simulink model "Final_V620140905h5b_fuben1"  (Simulink 7.9)
settings: Solver=FixedStepDiscrete  StartTime=0.0  StopTime=1  FixedStep=Auto  RelTol=1e-3
undefined symbols (not defined in the file or in its folder): Down, Up
libraries: tiiqmathlib x157, idelinklib_common x83, c2833xlib x37, simulink x12, c28xdmclib x12, c280xlib x7, simulink_extras x4, commutil2 x2, idelinklib_tgtpref x1, idelinklib_ticcs x1
(part 5 of 7)

== system Final_V620140905h5b_fuben1/Function-Call Subsystem1/RC filter2 ==
  x : Inport
  Constant2 : Constant  Value=a  OutDataTypeStr=fixdt(1,32,16)
  Constant3 : Constant  Value=1-a  OutDataTypeStr=fixdt(1,32,16)
  IQN x IQN : tiiqmathlib/IQN x IQN  multiplyOption=Multiply
  IQN x IQN1 : tiiqmathlib/IQN x IQN  multiplyOption=Multiply
  Sum2 : Sum
  Unit Delay2 : UnitDelay  SampleTime=-1
  y : Outport
  wires:
  x/1 -> IQN x IQN/1
  Constant2/1 -> IQN x IQN/2
  Constant3/1 -> IQN x IQN1/1
  IQN x IQN/1 -> Sum2/1
  IQN x IQN1/1 -> Sum2/2
  Sum2/1 -> y/1, Unit Delay2/1
  Unit Delay2/1 -> IQN x IQN1/2

== system Final_V620140905h5b_fuben1/Function-Call Subsystem1/RC filter3 ==
  x : Inport
  Constant2 : Constant  Value=a  OutDataTypeStr=Inherit: Inherit via back propagation
  Constant3 : Constant  Value=1-a  OutDataTypeStr=Inherit: Inherit via back propagation
  IQN x IQN : tiiqmathlib/IQN x IQN  multiplyOption=Multiply
  IQN x IQN1 : tiiqmathlib/IQN x IQN  multiplyOption=Multiply
  Sum2 : Sum
  Unit Delay2 : UnitDelay  SampleTime=-1
  y : Outport
  wires:
  Unit Delay2/1 -> IQN x IQN1/2
  Sum2/1 -> Unit Delay2/1, y/1
  IQN x IQN1/1 -> Sum2/2
  IQN x IQN/1 -> Sum2/1
  Constant3/1 -> IQN x IQN1/1
  Constant2/1 -> IQN x IQN/2
  x/1 -> IQN x IQN/1

== system Final_V620140905h5b_fuben1/Function-Call Subsystem1/RC filter4 ==
  x : Inport
  Constant2 : Constant  Value=a  OutDataTypeStr=Inherit: Inherit via back propagation
  Constant3 : Constant  Value=1-a  OutDataTypeStr=Inherit: Inherit via back propagation
  IQN x IQN : tiiqmathlib/IQN x IQN  multiplyOption=Multiply
  IQN x IQN1 : tiiqmathlib/IQN x IQN  multiplyOption=Multiply
  Sum2 : Sum
  Unit Delay2 : UnitDelay  SampleTime=-1
  y : Outport
  wires:
  x/1 -> IQN x IQN/1
  Constant2/1 -> IQN x IQN/2
  Constant3/1 -> IQN x IQN1/1
  IQN x IQN/1 -> Sum2/1
  IQN x IQN1/1 -> Sum2/2
  Sum2/1 -> y/1, Unit Delay2/1
  Unit Delay2/1 -> IQN x IQN1/2

== system Final_V620140905h5b_fuben1/Function-Call Subsystem1/RC filter9 ==
  x : Inport
  Constant2 : Constant  Value=a  OutDataTypeStr=fixdt(1,32,16)
  Constant3 : Constant  Value=1-a  OutDataTypeStr=fixdt(1,32,16)
  IQN x IQN : tiiqmathlib/IQN x IQN  multiplyOption=Multiply
  IQN x IQN1 : tiiqmathlib/IQN x IQN  multiplyOption=Multiply
  Sum2 : Sum
  Unit Delay2 : UnitDelay  SampleTime=-1
  y : Outport
  wires:
  Unit Delay2/1 -> IQN x IQN1/2
  Sum2/1 -> Unit Delay2/1, y/1
  IQN x IQN1/1 -> Sum2/2
  IQN x IQN/1 -> Sum2/1
  Constant3/1 -> IQN x IQN1/1
  Constant2/1 -> IQN x IQN/2
  x/1 -> IQN x IQN/1

== system Final_V620140905h5b_fuben1/Function-Call Subsystem1/Soft-start1 ==
  Reset : Inport
  Constant29 : Constant  Value=a  OutDataTypeStr=fixdt(1,32,16)
  Integration 0 to maximal1 : Subsystem
  Vref : Outport
  wires:
  Reset/1 -> Integration 0 to maximal1/2(Reset)
  Integration 0 to maximal1/1(y) -> Vref/1
  Constant29/1 -> Integration 0 to maximal1/1(x)

== system Final_V620140905h5b_fuben1/Function-Call Subsystem1/Soft-start2 ==
  Reset : Inport
  Constant29 : Constant  Value=a  OutDataTypeStr=fixdt(1,32,16)
  Integration 0 to maximal1 : Subsystem
  Vref : Outport
  wires:
  Constant29/1 -> Integration 0 to maximal1/1(x)
  Integration 0 to maximal1/1(y) -> Vref/1
  Reset/1 -> Integration 0 to maximal1/2(Reset)

== system Final_V620140905h5b_fuben1/Function-Call Subsystem1/Soft-start4 ==
  Reset : Inport
  T : Inport  Port=2
  Constant9 : Constant  Value=0.01  OutDataTypeStr=fixdt(1,32,16)
  IQN / IQN : tiiqmathlib/IQN // IQN
  Integration 0 to maximal1 : Subsystem
  Vref : Outport
  wires:
  Reset/1 -> Integration 0 to maximal1/2(Reset)
  Integration 0 to maximal1/1(y) -> Vref/1
  Constant9/1 -> IQN / IQN/1
  IQN / IQN/1 -> Integration 0 to maximal1/1(x)
  T/1 -> IQN / IQN/2

== system Final_V620140905h5b_fuben1/Function-Call Subsystem1/Soft-start5 ==
  Reset : Inport
  Constant29 : Constant  Value=a  OutDataTypeStr=fixdt(1,32,16)
  Integration 0 to maximal1 : Subsystem
  Vref : Outport
  wires:
  Reset/1 -> Integration 0 to maximal1/2(Reset)
  Integration 0 to maximal1/1(y) -> Vref/1
  Constant29/1 -> Integration 0 to maximal1/1(x)

== system Final_V620140905h5b_fuben1/Function-Call Subsystem1/Soft-start6 ==
  Reset : Inport
  Constant29 : Constant  Value=a  OutDataTypeStr=fixdt(1,32,16)
  Integration 0 to maximal1 : Subsystem
  Vref : Outport
  wires:
  Reset/1 -> Integration 0 to maximal1/2(Reset)
  Integration 0 to maximal1/1(y) -> Vref/1
  Constant29/1 -> Integration 0 to maximal1/1(x)

== system Final_V620140905h5b_fuben1/Function-Call Subsystem1/Soft_turn_off ==
  In : Inport
  Enable : Inport  Port=2
  Constant5 : Constant  Value=0.5  OutDataTypeStr=fixdt(1,32,16)
  Saturation1 : Saturate  UpperLimit=1000  LowerLimit=0  LinearizeAsGain=off  ZeroCross=off  OutDataTypeStr=fixdt(1,32,16)
  Sum1 : Sum  Inputs=+-
  Switch4 : Switch  Criteria=u2 > Threshold  SaturateOnIntegerOverflow=on  InputSameDT=on
  Switch5 : Switch  Criteria=u2 > Threshold  SaturateOnIntegerOverflow=on  InputSameDT=on
  Unit Delay2 : UnitDelay  SampleTime=-1
  Ref : Outport
  wires:
  In/1 -> Switch5/1, Switch4/1
  Switch4/1 -> Ref/1
  Constant5/1 -> Sum1/2
  Unit Delay2/1 -> Sum1/1
  Sum1/1 -> Switch5/3
  Switch5/1 -> Saturation1/1
  Enable/1 -> Switch5/2, Switch4/2
  Saturation1/1 -> Switch4/3, Unit Delay2/1

== system Final_V620140905h5b_fuben1/Function-Call Subsystem1/Soft_turn_on ==
  Enable : Inport
  Vdc : Inport  Port=2
  Compare To Constant2 : simulink/Logic and Bit Operations/Compare To Constant  relop=>  const=165*0.97/1.732  OutDataTypeStr=boolean
  Logical Operator5 : Logic  AllPortsSameDT=off  OutDataTypeStr=boolean
  Relay1 : Relay  OnSwitchValue=680  OffSwitchValue=650  OutDataTypeStr=Inherit: Inherit via back propagation
  Sum16 : Sum
  Voltage soft start (from 0 to 1 within 10s)1 : Subsystem  mask{a=10, b=401/1.732, c=0}
      mask prompts: a "soft time"; b "max limit"; c "min limit"
  Voltage soft start (from 0 to 120 within 5s) : Subsystem  mask{a=10, b=165/1.732, c=0}
      mask prompts: a "soft time"; b "max limit"; c "min limit"
  Out : Outport
  wires:
  Voltage soft start (from 0 to 120 within 5s)/1(k) -> Sum16/1, Compare To Constant2/1
  Enable/1 -> Voltage soft start (from 0 to 120 within 5s)/1(Reset)
  Sum16/1 -> Out/1
  Vdc/1 -> Relay1/1
  Compare To Constant2/1 -> Logical Operator5/1
  Voltage soft start (from 0 to 1 within 10s)1/1(k) -> Sum16/2
  Logical Operator5/1 -> Voltage soft start (from 0 to 1 within 10s)1/1(Reset)
  Relay1/1 -> Logical Operator5/2

== system Final_V620140905h5b_fuben1/Function-Call Subsystem1/Subsystem ==
  Trig : Inport
  x : Inport  Port=2
  Constant11 : Constant  Value=30  OutDataTypeStr=fixdt(1,32,16)
  Constant7 : Constant  Value=50  OutDataTypeStr=fixdt(1,32,16)
  Relational Operator1 : RelationalOperator
  Relational Operator2 : RelationalOperator  Operator=<=
  Saturation2 : Saturate  UpperLimit=500  LowerLimit=-500  LinearizeAsGain=off  ZeroCross=off  OutDataTypeStr=fixdt(1,32,16)
  Triggered Subsystem1 : Subsystem  TreatAsAtomicUnit=on
  sample per n times : Subsystem  mask{n=200*10}
      mask prompts: n "Counter time n"
  On/off : Outport
  sum : Outport  Port=2
  wires:
  Constant11/1 -> Relational Operator1/1
  sample per n times/1(sum) -> Saturation2/1
  Triggered Subsystem1/1(Count1) -> Relational Operator2/2
  Constant7/1 -> Relational Operator2/1
  Relational Operator1/1 -> Triggered Subsystem1/1(Reset1)
  Trig/1 -> Triggered Subsystem1/Trigger
  Relational Operator2/1 -> On/off/1
  x/1 -> sample per n times/1(x)
  Saturation2/1 -> Relational Operator1/2, sum/1

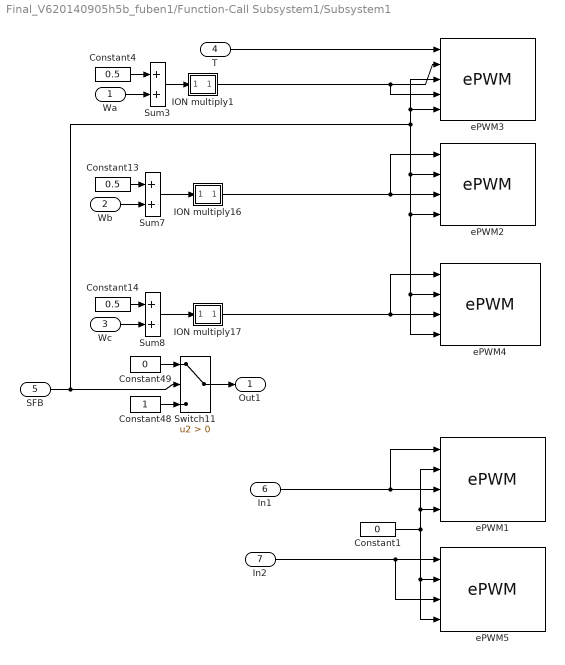
== system Final_V620140905h5b_fuben1/Function-Call Subsystem1/Subsystem1 ==
  Wa : Inport
  Wb : Inport  Port=2
  Wc : Inport  Port=3
  T : Inport  Port=4
  SFB : Inport  Port=5
  In1 : Inport  Port=6
  In2 : Inport  Port=7
  Constant1 : Constant  Value=0  OutDataTypeStr=fixdt(1,32,16)
  Constant13 : Constant  Value=0.5  OutDataTypeStr=fixdt(1,32,16)
  Constant14 : Constant  Value=0.5  OutDataTypeStr=fixdt(1,32,16)
  Constant4 : Constant  Value=0.5  OutDataTypeStr=fixdt(1,32,16)
  Constant48 : Constant  OutDataTypeStr=int16
  Constant49 : Constant  Value=0  OutDataTypeStr=int16
  ION multiply1 : Subsystem  mask{x=95}
      mask prompts: x "gain"
  ION multiply16 : Subsystem  mask{x=95}
      mask prompts: x "gain"
  ION multiply17 : Subsystem  mask{x=95}
      mask prompts: x "gain"
  Sum3 : Sum
  Sum7 : Sum
  Sum8 : Sum
  Switch11 : Switch  Criteria=u2 > Threshold  SaturateOnIntegerOverflow=on  InputSameDT=on
  ePWM1 : c280xlib/ePWM  checkMode=off  useModule=ePWM1  periodUnits=Clock cycles  timerSource=Specify via dialog  timerPeriod_clk=3750  timerPeriod_sec=1/20000  countingMode=Up-Down  synchronizationOption=Disable  synchronizationEnable=off  phaseActiveEnable=Disable  phaseDirection=Count down after sync  phaseActive=0  clockPrescale=1  HSclockPrescale=1  ePWMxAStatus=off  CMPAUnits=Percentages  CMPASource=Input port  CMPAValue_per=0  CMPAValue_clk=32000  ePWMxAactionLogic1=Do nothing  ePWMxAactionLogic2=Do nothing  ePWMxAactionLogic3=Clear  ePWMxAactionLogic4=Set  ePWMxAactionLogic5=Do nothing  ePWMxAactionLogic6=Do nothing  ePWMxALoadMode=Load on CTR=Zero  ePWMxACSFenable=on  ePWMxACSFvalue=Forcing Disable  ePWMxASFreload=Zero  enHRPWM=off  HRPWM_LoadMode=CTR=ZERO  HRPWM_CTLMode=Phase control mode  HRPWM_EDGMode=Both edge  enSFO=on  ePWMxBStatus=on  CMPBUnits=Percentages  CMPBSource=Input port  CMPBValue_per=0  CMPBValue_clk=32000  ePWMxBactionLogic1=Do nothing  ePWMxBactionLogic2=Do nothing  ePWMxBactionLogic3=Do nothing  ePWMxBactionLogic4=Do nothing  ePWMxBactionLogic5=Set  ePWMxBactionLogic6=Clear  ePWMxBLoadMode=Load on CTR=Zero  ePWMxBCSFenable=on  ePWMxBCSFvalue=Forcing Disable  ePWMxBSFreload=Zero  enableDBePWMxA=on  enableDBePWMxB=on  DBpolarity=ALC  DBedgeDelay=Positive  DBSource_ePWMxA=ePWMxB  DBSource_ePWMxB=ePWMxB  DBperiodSource=Specify via dialog  REDperiod=300  FEDperiod=300  adcstartModuleA=off  adcrequestEventA=First event  adcstartEventA=CTR=Zero  adcstartModuleB=off  adcrequestEventB=First event  adcstartEventB=CTR=Zero  intEn=off  intPrd=First event  intSel=CTR=Zero  chopperEnable=off  chopperFrequency=1  chopperFirstwidth=1  chopperDuty=12.5%  tripZonesource=Specify via dialog  tzselOSHT1=off  tzselOSHT2=off  tzselOSHT3=off  tzselOSHT4=off  tzselOSHT5=off  tzselOSHT6=off  tzselCBC1=off  tzselCBC2=off  tzselCBC3=off  tzselCBC4=off  tzselCBC5=off  tzselCBC6=off  enTzOstIntr=off  enTzCbcIntr=off  ePWMxAforced=No action  ePWMxBforced=No action  timerPeriod=-1  ePWMxAValue=0  ePWMxBValue=0  tripZoneoption=OSHT
  ePWM2 : c280xlib/ePWM  checkMode=off  useModule=ePWM5  periodUnits=Clock cycles  timerSource=Specify via dialog  timerPeriod_clk=15000  timerPeriod_sec=1/20000  countingMode=Up-Down  synchronizationOption=Disable  synchronizationEnable=off  phaseActiveEnable=Disable  phaseDirection=Count down after sync  phaseActive=0  clockPrescale=1  HSclockPrescale=1  ePWMxAStatus=off  CMPAUnits=Percentages  CMPASource=Input port  CMPAValue_per=0  CMPAValue_clk=32000  ePWMxAactionLogic1=Do nothing  ePWMxAactionLogic2=Do nothing  ePWMxAactionLogic3=Clear  ePWMxAactionLogic4=Set  ePWMxAactionLogic5=Do nothing  ePWMxAactionLogic6=Do nothing  ePWMxALoadMode=Load on CTR=Zero  ePWMxACSFenable=on  ePWMxACSFvalue=Forcing Disable  ePWMxASFreload=Zero  enHRPWM=off  HRPWM_LoadMode=CTR=ZERO  HRPWM_CTLMode=Phase control mode  HRPWM_EDGMode=Both edge  enSFO=on  ePWMxBStatus=on  CMPBUnits=Percentages  CMPBSource=Input port  CMPBValue_per=0  CMPBValue_clk=32000  ePWMxBactionLogic1=Do nothing  ePWMxBactionLogic2=Do nothing  ePWMxBactionLogic3=Do nothing  ePWMxBactionLogic4=Do nothing  ePWMxBactionLogic5=Set  ePWMxBactionLogic6=Clear  ePWMxBLoadMode=Load on CTR=Zero  ePWMxBCSFenable=on  ePWMxBCSFvalue=Forcing Disable  ePWMxBSFreload=Zero  enableDBePWMxA=on  enableDBePWMxB=on  DBpolarity=ALC  DBedgeDelay=Positive  DBSource_ePWMxA=ePWMxB  DBSource_ePWMxB=ePWMxB  DBperiodSource=Specify via dialog  REDperiod=300  FEDperiod=300  adcstartModuleA=off  adcrequestEventA=First event  adcstartEventA=CTR=Zero  adcstartModuleB=off  adcrequestEventB=First event  adcstartEventB=CTR=Zero  intEn=off  intPrd=First event  intSel=CTR=Zero  chopperEnable=off  chopperFrequency=1  chopperFirstwidth=1  chopperDuty=12.5%  tripZonesource=Specify via dialog  tzselOSHT1=off  tzselOSHT2=off  tzselOSHT3=off  tzselOSHT4=off  tzselOSHT5=off  tzselOSHT6=off  tzselCBC1=off  tzselCBC2=off  tzselCBC3=off  tzselCBC4=off  tzselCBC5=off  tzselCBC6=off  enTzOstIntr=off  enTzCbcIntr=off  ePWMxAforced=No action  ePWMxBforced=No action  timerPeriod=-1  ePWMxAValue=0  ePWMxBValue=0  tripZoneoption=OSHT
  ePWM3 : c280xlib/ePWM  checkMode=off  useModule=ePWM4  periodUnits=Clock cycles  timerSource=Input port  timerPeriod_clk=15000  timerPeriod_sec=1/20000  countingMode=Up-Down  synchronizationOption=Disable  synchronizationEnable=off  phaseActiveEnable=Disable  phaseDirection=Count down after sync  phaseActive=0  clockPrescale=1  HSclockPrescale=1  ePWMxAStatus=off  CMPAUnits=Percentages  CMPASource=Input port  CMPAValue_per=0  CMPAValue_clk=32000  ePWMxAactionLogic1=Do nothing  ePWMxAactionLogic2=Do nothing  ePWMxAactionLogic3=Clear  ePWMxAactionLogic4=Set  ePWMxAactionLogic5=Do nothing  ePWMxAactionLogic6=Do nothing  ePWMxALoadMode=Load on CTR=Zero  ePWMxACSFenable=on  ePWMxACSFvalue=Forcing Disable  ePWMxASFreload=Zero  enHRPWM=off  HRPWM_LoadMode=CTR=ZERO  HRPWM_CTLMode=Phase control mode  HRPWM_EDGMode=Both edge  enSFO=on  ePWMxBStatus=on  CMPBUnits=Percentages  CMPBSource=Input port  CMPBValue_per=0  CMPBValue_clk=32000  ePWMxBactionLogic1=Do nothing  ePWMxBactionLogic2=Do nothing  ePWMxBactionLogic3=Do nothing  ePWMxBactionLogic4=Do nothing  ePWMxBactionLogic5=Set  ePWMxBactionLogic6=Clear  ePWMxBLoadMode=Load on CTR=Zero  ePWMxBCSFenable=on  ePWMxBCSFvalue=Forcing Disable  ePWMxBSFreload=Zero  enableDBePWMxA=on  enableDBePWMxB=on  DBpolarity=ALC  DBedgeDelay=Positive  DBSource_ePWMxA=ePWMxB  DBSource_ePWMxB=ePWMxB  DBperiodSource=Specify via dialog  REDperiod=300  FEDperiod=300  adcstartModuleA=off  adcrequestEventA=First event  adcstartEventA=CTR=Zero  adcstartModuleB=off  adcrequestEventB=First event  adcstartEventB=CTR=Zero  intEn=on  intPrd=First event  intSel=CTR=Zero  chopperEnable=off  chopperFrequency=1  chopperFirstwidth=1  chopperDuty=12.5%  tripZonesource=Specify via dialog  tzselOSHT1=off  tzselOSHT2=off  tzselOSHT3=off  tzselOSHT4=off  tzselOSHT5=off  tzselOSHT6=off  tzselCBC1=off  tzselCBC2=off  tzselCBC3=off  tzselCBC4=off  tzselCBC5=off  tzselCBC6=off  enTzOstIntr=off  enTzCbcIntr=off  ePWMxAforced=No action  ePWMxBforced=No action  timerPeriod=-1  ePWMxAValue=0  ePWMxBValue=0  tripZoneoption=OSHT
  ePWM4 : c280xlib/ePWM  checkMode=off  useModule=ePWM6  periodUnits=Clock cycles  timerSource=Specify via dialog  timerPeriod_clk=15000  timerPeriod_sec=1/20000  countingMode=Up-Down  synchronizationOption=Disable  synchronizationEnable=off  phaseActiveEnable=Disable  phaseDirection=Count down after sync  phaseActive=0  clockPrescale=1  HSclockPrescale=1  ePWMxAStatus=off  CMPAUnits=Percentages  CMPASource=Input port  CMPAValue_per=0  CMPAValue_clk=32000  ePWMxAactionLogic1=Do nothing  ePWMxAactionLogic2=Do nothing  ePWMxAactionLogic3=Clear  ePWMxAactionLogic4=Set  ePWMxAactionLogic5=Do nothing  ePWMxAactionLogic6=Do nothing  ePWMxALoadMode=Load on CTR=Zero  ePWMxACSFenable=on  ePWMxACSFvalue=Forcing Disable  ePWMxASFreload=Zero  enHRPWM=off  HRPWM_LoadMode=CTR=ZERO  HRPWM_CTLMode=Phase control mode  HRPWM_EDGMode=Both edge  enSFO=on  ePWMxBStatus=on  CMPBUnits=Percentages  CMPBSource=Input port  CMPBValue_per=0  CMPBValue_clk=32000  ePWMxBactionLogic1=Do nothing  ePWMxBactionLogic2=Do nothing  ePWMxBactionLogic3=Do nothing  ePWMxBactionLogic4=Do nothing  ePWMxBactionLogic5=Set  ePWMxBactionLogic6=Clear  ePWMxBLoadMode=Load on CTR=Zero  ePWMxBCSFenable=on  ePWMxBCSFvalue=Forcing Disable  ePWMxBSFreload=Zero  enableDBePWMxA=on  enableDBePWMxB=on  DBpolarity=ALC  DBedgeDelay=Positive  DBSource_ePWMxA=ePWMxB  DBSource_ePWMxB=ePWMxB  DBperiodSource=Specify via dialog  REDperiod=300  FEDperiod=300  adcstartModuleA=off  adcrequestEventA=First event  adcstartEventA=CTR=Zero  adcstartModuleB=off  adcrequestEventB=First event  adcstartEventB=CTR=Zero  intEn=off  intPrd=First event  intSel=CTR=Zero  chopperEnable=off  chopperFrequency=1  chopperFirstwidth=1  chopperDuty=12.5%  tripZonesource=Specify via dialog  tzselOSHT1=off  tzselOSHT2=off  tzselOSHT3=off  tzselOSHT4=off  tzselOSHT5=off  tzselOSHT6=off  tzselCBC1=off  tzselCBC2=off  tzselCBC3=off  tzselCBC4=off  tzselCBC5=off  tzselCBC6=off  enTzOstIntr=off  enTzCbcIntr=off  ePWMxAforced=No action  ePWMxBforced=No action  timerPeriod=-1  ePWMxAValue=0  ePWMxBValue=0  tripZoneoption=OSHT
  ePWM5 : c280xlib/ePWM  checkMode=off  useModule=ePWM2  periodUnits=Clock cycles  timerSource=Specify via dialog  timerPeriod_clk=3750  timerPeriod_sec=1/20000  countingMode=Up-Down  synchronizationOption=Disable  synchronizationEnable=off  phaseActiveEnable=Disable  phaseDirection=Count down after sync  phaseActive=0  clockPrescale=1  HSclockPrescale=1  ePWMxAStatus=off  CMPAUnits=Percentages  CMPASource=Input port  CMPAValue_per=0  CMPAValue_clk=32000  ePWMxAactionLogic1=Do nothing  ePWMxAactionLogic2=Do nothing  ePWMxAactionLogic3=Clear  ePWMxAactionLogic4=Set  ePWMxAactionLogic5=Do nothing  ePWMxAactionLogic6=Do nothing  ePWMxALoadMode=Load on CTR=Zero  ePWMxACSFenable=on  ePWMxACSFvalue=Forcing Disable  ePWMxASFreload=Zero  enHRPWM=off  HRPWM_LoadMode=CTR=ZERO  HRPWM_CTLMode=Phase control mode  HRPWM_EDGMode=Both edge  enSFO=on  ePWMxBStatus=on  CMPBUnits=Percentages  CMPBSource=Input port  CMPBValue_per=0  CMPBValue_clk=32000  ePWMxBactionLogic1=Do nothing  ePWMxBactionLogic2=Do nothing  ePWMxBactionLogic3=Do nothing  ePWMxBactionLogic4=Do nothing  ePWMxBactionLogic5=Set  ePWMxBactionLogic6=Clear  ePWMxBLoadMode=Load on CTR=Zero  ePWMxBCSFenable=on  ePWMxBCSFvalue=Forcing Disable  ePWMxBSFreload=Zero  enableDBePWMxA=on  enableDBePWMxB=on  DBpolarity=ALC  DBedgeDelay=Positive  DBSource_ePWMxA=ePWMxB  DBSource_ePWMxB=ePWMxB  DBperiodSource=Specify via dialog  REDperiod=300  FEDperiod=300  adcstartModuleA=off  adcrequestEventA=First event  adcstartEventA=CTR=Zero  adcstartModuleB=off  adcrequestEventB=First event  adcstartEventB=CTR=Zero  intEn=off  intPrd=First event  intSel=CTR=Zero  chopperEnable=off  chopperFrequency=1  chopperFirstwidth=1  chopperDuty=12.5%  tripZonesource=Specify via dialog  tzselOSHT1=off  tzselOSHT2=off  tzselOSHT3=off  tzselOSHT4=off  tzselOSHT5=off  tzselOSHT6=off  tzselCBC1=off  tzselCBC2=off  tzselCBC3=off  tzselCBC4=off  tzselCBC5=off  tzselCBC6=off  enTzOstIntr=off  enTzCbcIntr=off  ePWMxAforced=No action  ePWMxBforced=No action  timerPeriod=-1  ePWMxAValue=0  ePWMxBValue=0  tripZoneoption=OSHT
  Out1 : Outport
  wires:
  Constant4/1 -> Sum3/1
  Sum3/1 -> ION multiply1/1(x)
  Constant13/1 -> Sum7/1
  Sum7/1 -> ION multiply16/1(x)
  Constant14/1 -> Sum8/1
  Sum8/1 -> ION multiply17/1(x)
  ION multiply1/1(Kx) -> ePWM3/4, ePWM3/2
  ION multiply16/1(Kx) -> ePWM2/1, ePWM2/3
  ION multiply17/1(Kx) -> ePWM4/3, ePWM4/1
  SFB/1 -> Switch11/2, ePWM4/4, ePWM4/2, ePWM2/4, ePWM2/2, ePWM3/5, ePWM3/3
  Constant48/1 -> Switch11/3
  Constant49/1 -> Switch11/1
  T/1 -> ePWM3/1
  Wa/1 -> Sum3/2
  Wb/1 -> Sum7/2
  Wc/1 -> Sum8/2
  Switch11/1 -> Out1/1
  In1/1 -> ePWM1/1, ePWM1/3
  In2/1 -> ePWM5/1, ePWM5/3
  Constant1/1 -> ePWM1/4, ePWM1/2, ePWM5/2, ePWM5/4

== system Final_V620140905h5b_fuben1/Function-Call Subsystem1/Subsystem2 ==
  In1 : Inport
  In2 : Inport  Port=2
  IQN x IQN2 : tiiqmathlib/IQN x IQN  multiplyOption=Multiply
  IQN x IQN3 : tiiqmathlib/IQN x IQN  multiplyOption=Multiply
  Square Root IQN : tiiqmathlib/Square Root IQN  functionOption=Square root
  Sum17 : Sum
  Out1 : Outport
  wires:
  IQN x IQN2/1 -> Sum17/1
  IQN x IQN3/1 -> Sum17/2
  Sum17/1 -> Square Root IQN/1
  In1/1 -> IQN x IQN2/1, IQN x IQN2/2
  In2/1 -> IQN x IQN3/1, IQN x IQN3/2
  Square Root IQN/1 -> Out1/1

== system Final_V620140905h5b_fuben1/Function-Call Subsystem1/Subsystem8 ==
  fre : Inport
  1 : Constant  Value=5000  OutDataTypeStr=Inherit: Inherit via back propagation
  10 : Constant  Value=5000  OutDataTypeStr=Inherit: Inherit via back propagation
  2 : Constant  Value=5000  OutDataTypeStr=Inherit: Inherit via back propagation
  Sum5 : Sum
  Sum6 : Sum  Inputs=+-
  Sum7 : Sum  Inputs=+-
  Sum8 : Sum
  Switch1 : Switch  Criteria=u2 > Threshold  SaturateOnIntegerOverflow=on  InputSameDT=on
  Switch10 : Switch  Criteria=u2 > Threshold  SaturateOnIntegerOverflow=on  InputSameDT=on
  Unit Delay5 : UnitDelay  SampleTime=-1
  angle : Outport
  wires:
  fre/1 -> Sum5/2
  Switch10/1 -> angle/1, Unit Delay5/1
  2/1 -> Sum8/2
  Sum8/1 -> Switch10/3
  Switch1/1 -> Switch10/1, Sum8/1, Switch10/2
  Sum7/1 -> Switch1/1
  1/1 -> Sum7/2
  Sum6/1 -> Switch1/2
  10/1 -> Sum6/2
  Sum5/1 -> Sum7/1, Sum6/1, Switch1/3
  Unit Delay5/1 -> Sum5/1

== system Final_V620140905h5b_fuben1/Function-Call Subsystem1/Vdc_protect ==
  Reset : Inport
  Vdin : Inport  Port=2
  Constant16 : Constant  Value=0  OutDataTypeStr=boolean
  Constant19 : Constant  Value=0  OutDataTypeStr=fixdt(1,32,16)
  Constant20 : Constant  OutDataTypeStr=fixdt(1,32,16)
  Constant50 : Constant  Value=780  OutDataTypeStr=fixdt(1,32,16)
  Constant9 : Constant  Value=650  OutDataTypeStr=fixdt(1,32,16)
  IQN x IQN : tiiqmathlib/IQN x IQN  multiplyOption=Multiply
  Logical Operator8 : Logic  Operator=OR  AllPortsSameDT=off  OutDataTypeStr=boolean
  Relational Operator1 : RelationalOperator  Operator=<  OutDataTypeStr=boolean
  Relational Operator4 : RelationalOperator  Operator=>  OutDataTypeStr=boolean
  Relay1 : Relay  OnSwitchValue=660  OffSwitchValue=50
  S-R Flip-Flop2 : simulink_extras/Flip Flops/S-R Flip-Flop  initial_condition=0
  Switch6 : Switch  Criteria=u2 > Threshold  SaturateOnIntegerOverflow=on  InputSameDT=on
  Switch7 : Switch  Criteria=u2 > Threshold  SaturateOnIntegerOverflow=on  InputSameDT=on
  Terminator1 : Terminator
  Vdguoya : Outport
  wires:
  Constant50/1 -> Relational Operator4/2
  Constant9/1 -> Relational Operator1/2
  Relational Operator4/1 -> Logical Operator8/1
  Relational Operator1/1 -> Logical Operator8/2
  Logical Operator8/1 -> Switch6/1
  Relay1/1 -> Switch6/2
  Constant16/1 -> Switch6/3
  Switch6/1 -> S-R Flip-Flop2/1
  Vdin/1 -> Relational Operator4/1, Relational Operator1/1, IQN x IQN/1
  S-R Flip-Flop2/2 -> Terminator1/1
  S-R Flip-Flop2/1 -> Vdguoya/1
  Reset/1 -> Switch7/2, S-R Flip-Flop2/2
  Constant19/1 -> Switch7/1
  Constant20/1 -> Switch7/3
  Switch7/1 -> IQN x IQN/2
  IQN x IQN/1 -> Relay1/1

== system Final_V620140905h5b_fuben1/Function-Call Subsystem1/Voltage protect ==
  V1 : Inport
  Reset : Inport  Port=2
  Constant19 : Constant  Value=0  OutDataTypeStr=boolean
  Constant20 : Constant  OutDataTypeStr=boolean
  RC filter11 : Subsystem  mask{a=0.1}
      mask prompts: a "Time Constant"
  S-R Flip-Flop4 : simulink_extras/Flip Flops/S-R Flip-Flop  initial_condition=0
  Switch6 : Switch  Criteria=u2 > Threshold  Threshold=400*1.414/1.732*1.5  SaturateOnIntegerOverflow=on  InputSameDT=on
  Terminator3 : Terminator
  softwave_V : Outport
  wires:
  RC filter11/1(y) -> Switch6/2
  S-R Flip-Flop4/2 -> Terminator3/1
  Reset/1 -> S-R Flip-Flop4/2
  S-R Flip-Flop4/1 -> softwave_V/1
  Switch6/1 -> S-R Flip-Flop4/1
  Constant19/1 -> Switch6/3
  Constant20/1 -> Switch6/1
  V1/1 -> RC filter11/1(x)

== system Final_V620140905h5b_fuben1/Function-Call Subsystem1/abc/dq-grid voltage1 ==
  Uga : Inport
  Ugb : Inport  Port=2
  Arctangent IQN1 : tiiqmathlib/Arctangent IQN  tanOption=atan2PU (per unit)
  Clarke : c28xdmclib/Clarke Transformation
  Constant26 : Constant  Value=0.03886  OutDataTypeStr=fixdt(1,32,16)
  Park : c28xdmclib/Park Transformation
  RC filter1 : Subsystem  mask{a=0.2}
      mask prompts: a "Time Constant"
  RC filter5 : Subsystem  mask{a=0.2}
      mask prompts: a "Time Constant"
  Sum9 : Sum
  Ugd : Outport
  Ugq : Outport  Port=2
  Phase : Outport  Port=3
  wires:
  Sum9/1 -> Park/3, Phase/1
  Constant26/1 -> Sum9/2
  Arctangent IQN1/1 -> Sum9/1
  RC filter1/1(y) -> Arctangent IQN1/2
  RC filter5/1(y) -> Arctangent IQN1/1
  Clarke/1 -> RC filter5/1(x), Park/1
  Clarke/2 -> RC filter1/1(x), Park/2
  Park/1 -> Ugd/1
  Uga/1 -> Clarke/1
  Park/2 -> Ugq/1
  Ugb/1 -> Clarke/2

== system Final_V620140905h5b_fuben1/Function-Call Subsystem1/abc/dq-grid voltage3 ==
  iga : Inport
  igb : Inport  Port=2
  angle : Inport  Port=3
  Clarke : c28xdmclib/Clarke Transformation
  Park : c28xdmclib/Park Transformation
  igd : Outport
  igq : Outport  Port=2
  wires:
  angle/1 -> Park/3
  Clarke/1 -> Park/1
  Clarke/2 -> Park/2
  Park/1 -> igd/1
  iga/1 -> Clarke/1
  Park/2 -> igq/1
  igb/1 -> Clarke/2

== system Final_V620140905h5b_fuben1/Function-Call Subsystem1/abc/dq-grid voltage4 ==
  iga : Inport
  igb : Inport  Port=2
  angle : Inport  Port=3
  Clarke : c28xdmclib/Clarke Transformation
  Park : c28xdmclib/Park Transformation
  igd : Outport
  igq : Outport  Port=2
  wires:
  angle/1 -> Park/3
  Clarke/1 -> Park/1
  Clarke/2 -> Park/2
  Park/1 -> igd/1
  iga/1 -> Clarke/1
  Park/2 -> igq/1
  igb/1 -> Clarke/2

== system Final_V620140905h5b_fuben1/Function-Call Subsystem1/abc/dq-grid voltage5 ==
  iga : Inport
  igb : Inport  Port=2
  angle : Inport  Port=3
  Clarke : c28xdmclib/Clarke Transformation
  ION multiply17 : Subsystem  mask{x=-1}
      mask prompts: x "gain"
  Park : c28xdmclib/Park Transformation
  igd : Outport
  igq : Outport  Port=2
  wires:
  igb/1 -> Clarke/2
  Park/2 -> ION multiply17/1(x)
  iga/1 -> Clarke/1
  Park/1 -> igd/1
  Clarke/2 -> Park/2
  Clarke/1 -> Park/1
  angle/1 -> Park/3
  ION multiply17/1(Kx) -> igq/1

== system Final_V620140905h5b_fuben1/Function-Call Subsystem1/abc/dq-grid voltage7 ==
  Uga : Inport
  Ugb : Inport  Port=2
  Arctangent IQN1 : tiiqmathlib/Arctangent IQN  tanOption=atan2PU (per unit)
  Clarke : c28xdmclib/Clarke Transformation
  Constant26 : Constant  Value=0.03886  OutDataTypeStr=fixdt(1,32,16)
  Park : c28xdmclib/Park Transformation
  RC filter1 : Subsystem  mask{a=0.2}
      mask prompts: a "Time Constant"
  RC filter5 : Subsystem  mask{a=0.2}
      mask prompts: a "Time Constant"
  Sum9 : Sum
  Ugd : Outport
  Ugq : Outport  Port=2
  Phase : Outport  Port=3
  wires:
  Ugb/1 -> Clarke/2
  Park/2 -> Ugq/1
  Uga/1 -> Clarke/1
  Park/1 -> Ugd/1
  Clarke/2 -> Park/2, RC filter1/1(x)
  Clarke/1 -> Park/1, RC filter5/1(x)
  RC filter5/1(y) -> Arctangent IQN1/1
  RC filter1/1(y) -> Arctangent IQN1/2
  Arctangent IQN1/1 -> Sum9/1
  Constant26/1 -> Sum9/2
  Sum9/1 -> Phase/1, Park/3

== system Final_V620140905h5b_fuben1/Function-Call Subsystem1/set and reset ==
  In1 : Inport
  Compare To Constant3 : simulink/Logic and Bit Operations/Compare To Constant  relop=>  const=50  OutDataTypeStr=boolean
  Compare To Constant4 : simulink/Logic and Bit Operations/Compare To Constant  relop=<  const=99  OutDataTypeStr=boolean
  Logical Operator12 : Logic  AllPortsSameDT=off  OutDataTypeStr=boolean
  Logical Operator14 : Logic  Operator=OR  AllPortsSameDT=off  OutDataTypeStr=boolean
  Logical Operator15 : Logic  Operator=NOT  Inputs=1  AllPortsSameDT=off  OutDataTypeStr=boolean
  Soft-start3 : Subsystem  mask{a=0.02/0.04, b=100}
      mask prompts: a "soft time"; b "Vref"
  Out1 : Outport
  wires:
  In1/1 -> Logical Operator14/2, Logical Operator15/1
  Logical Operator15/1 -> Soft-start3/1(Reset)
  Soft-start3/1(Vref) -> Compare To Constant3/1, Compare To Constant4/1
  Compare To Constant3/1 -> Logical Operator12/1
  Compare To Constant4/1 -> Logical Operator12/2
  Logical Operator12/1 -> Logical Operator14/1
  Logical Operator14/1 -> Out1/1

== system Final_V620140905h5b_fuben1/Function-Call Subsystem1/softwave and hardwave protect ==
  Over_V : Inport
  Over_Vdc : Inport  Port=2
  Over_I : Inport  Port=3
  Over_Ip : Inport  Port=4
  PWM : Inport  Port=5
  Constant27 : Constant  OutDataTypeStr=uint16
  Constant28 : Constant  OutDataTypeStr=uint16
  Constant9 : Constant  OutDataTypeStr=uint16
  Digital Input : c2833xlib/Digital Input  GPIO_Number=GPIO48~GPIO55  GPIO_Bit0=off  GPIO_Bit1=off  GPIO_Bit2=off  GPIO_Bit3=on  GPIO_Bit4=off  GPIO_Bit5=off  GPIO_Bit6=off  GPIO_Bit7=off  sampleTime=-1  dataType=uint16  GPIO_Bit0_Qualification=Sync to SYSCLKOUT  GPIO_Bit1_Qualification=Sync to SYSCLKOUT  GPIO_Bit2_Qualification=Sync to SYSCLKOUT  GPIO_Bit3_Qualification=Sync to SYSCLKOUT  GPIO_Bit4_Qualification=Sync to SYSCLKOUT  GPIO_Bit5_Qualification=Sync to SYSCLKOUT  GPIO_Bit6_Qualification=Sync to SYSCLKOUT  GPIO_Bit7_Qualification=Sync to SYSCLKOUT  Qualification_Period=-1
  Digital Input1 : c2833xlib/Digital Input  GPIO_Number=GPIO48~GPIO55  GPIO_Bit0=off  GPIO_Bit1=off  GPIO_Bit2=off  GPIO_Bit3=off  GPIO_Bit4=on  GPIO_Bit5=off  GPIO_Bit6=off  GPIO_Bit7=off  sampleTime=-1  dataType=uint16  GPIO_Bit0_Qualification=Sync to SYSCLKOUT  GPIO_Bit1_Qualification=Sync to SYSCLKOUT  GPIO_Bit2_Qualification=Sync to SYSCLKOUT  GPIO_Bit3_Qualification=Sync to SYSCLKOUT  GPIO_Bit4_Qualification=Sync to SYSCLKOUT  GPIO_Bit5_Qualification=Sync to SYSCLKOUT  GPIO_Bit6_Qualification=Sync to SYSCLKOUT  GPIO_Bit7_Qualification=Sync to SYSCLKOUT  Qualification_Period=-1
  Digital Input2 : c2833xlib/Digital Input  GPIO_Number=GPIO48~GPIO55  GPIO_Bit0=off  GPIO_Bit1=off  GPIO_Bit2=off  GPIO_Bit3=off  GPIO_Bit4=off  GPIO_Bit5=on  GPIO_Bit6=off  GPIO_Bit7=off  sampleTime=-1  dataType=uint16  GPIO_Bit0_Qualification=Sync to SYSCLKOUT  GPIO_Bit1_Qualification=Sync to SYSCLKOUT  GPIO_Bit2_Qualification=Sync to SYSCLKOUT  GPIO_Bit3_Qualification=Sync to SYSCLKOUT  GPIO_Bit4_Qualification=Sync to SYSCLKOUT  GPIO_Bit5_Qualification=Sync to SYSCLKOUT  GPIO_Bit6_Qualification=Sync to SYSCLKOUT  GPIO_Bit7_Qualification=Sync to SYSCLKOUT  Qualification_Period=-1
  Logical Operator1 : Logic  Operator=OR  AllPortsSameDT=off  OutDataTypeStr=boolean
  Logical Operator18 : Logic  Operator=OR  Inputs=7  AllPortsSameDT=off  OutDataTypeStr=boolean
  Relational Operator : RelationalOperator  Operator=>  OutDataTypeStr=boolean
  Relational Operator1 : RelationalOperator  Operator=>  OutDataTypeStr=boolean
  Relational Operator2 : RelationalOperator  Operator=>  OutDataTypeStr=boolean
  SFB : Outport
  protect singal : Outport  Port=2
  wires:
  Digital Input/1 -> Relational Operator/2
  Constant9/1 -> Relational Operator/1
  Digital Input1/1 -> Relational Operator1/2
  Constant27/1 -> Relational Operator1/1
  Digital Input2/1 -> Relational Operator2/2
  Constant28/1 -> Relational Operator2/1
  Logical Operator18/1 -> protect singal/1, Logical Operator1/1
  Over_V/1 -> Logical Operator18/5
  Over_Vdc/1 -> Logical Operator18/6
  Over_I/1 -> Logical Operator18/7
  Over_Ip/1 -> Logical Operator18/4
  Relational Operator/1 -> Logical Operator18/1
  Relational Operator2/1 -> Logical Operator18/3
  Relational Operator1/1 -> Logical Operator18/2
  PWM/1 -> Logical Operator1/2
  Logical Operator1/1 -> SFB/1

== system Final_V620140905h5b_fuben1/Function-Call Subsystem3/Integration 0 to maximal3 ==
  x : Inport
  3 : Constant  Value=a  OutDataTypeStr=fixdt(1,32,16)
  Relational Operator1 : RelationalOperator  Operator=<=
  Sum1 : Sum  Inputs=+-
  Sum2 : Sum
  Switch2 : Switch  Criteria=u2 > Threshold  SaturateOnIntegerOverflow=on  InputSameDT=on
  Unit Delay1 : UnitDelay  SampleTime=-1
  y : Outport
  Zero Trig : Outport  Port=2
  wires:
  x/1 -> Sum2/2
  Sum1/1 -> Switch2/3
  Switch2/1 -> y/1, Unit Delay1/1
  Relational Operator1/1 -> Zero Trig/1, Switch2/2
  3/1 -> Sum1/2, Relational Operator1/2
  Sum2/1 -> Sum1/1, Relational Operator1/1, Switch2/1
  Unit Delay1/1 -> Sum2/1

== system Final_V620140905h5b_fuben1/Subsystem1/ION multiply1 ==
  x : Inport
  Constant2 : Constant  Value=x  OutDataTypeStr=fixdt(1,32,16)
  IQN x IQN : tiiqmathlib/IQN x IQN  multiplyOption=Multiply
  Kx : Outport
  wires:
  Constant2/1 -> IQN x IQN/2
  x/1 -> IQN x IQN/1
  IQN x IQN/1 -> Kx/1

== system Final_V620140905h5b_fuben1/Subsystem1/ION multiply2 ==
  x : Inport
  Constant2 : Constant  Value=x  OutDataTypeStr=fixdt(1,32,16)
  IQN x IQN : tiiqmathlib/IQN x IQN  multiplyOption=Multiply
  Kx : Outport
  wires:
  IQN x IQN/1 -> Kx/1
  x/1 -> IQN x IQN/1
  Constant2/1 -> IQN x IQN/2

== system Final_V620140905h5b_fuben1/Subsystem1/ION multiply3 ==
  x : Inport
  Constant2 : Constant  Value=x  OutDataTypeStr=fixdt(1,32,16)
  IQN x IQN : tiiqmathlib/IQN x IQN  multiplyOption=Multiply
  Kx : Outport
  wires:
  Constant2/1 -> IQN x IQN/2
  x/1 -> IQN x IQN/1
  IQN x IQN/1 -> Kx/1

== system Final_V620140905h5b_fuben1/Subsystem1/ION multiply4 ==
  x : Inport
  Constant2 : Constant  Value=x  OutDataTypeStr=fixdt(1,32,16)
  IQN x IQN : tiiqmathlib/IQN x IQN  multiplyOption=Multiply
  Kx : Outport
  wires:
  IQN x IQN/1 -> Kx/1
  x/1 -> IQN x IQN/1
  Constant2/1 -> IQN x IQN/2

== system Final_V620140905h5b_fuben1/Subsystem1/ION multiply42 ==
  x : Inport
  Constant2 : Constant  Value=x  OutDataTypeStr=fixdt(1,32,16)
  IQN x IQN : tiiqmathlib/IQN x IQN  multiplyOption=Multiply
  Kx : Outport
  wires:
  IQN x IQN/1 -> Kx/1
  x/1 -> IQN x IQN/1
  Constant2/1 -> IQN x IQN/2

== system Final_V620140905h5b_fuben1/Subsystem1/ION multiply5 ==
  x : Inport
  Constant2 : Constant  Value=x  OutDataTypeStr=fixdt(1,32,16)
  IQN x IQN : tiiqmathlib/IQN x IQN  multiplyOption=Multiply
  Kx : Outport
  wires:
  IQN x IQN/1 -> Kx/1
  x/1 -> IQN x IQN/1
  Constant2/1 -> IQN x IQN/2

== system Final_V620140905h5b_fuben1/Subsystem1/ION multiply6 ==
  x : Inport
  Constant2 : Constant  Value=x  OutDataTypeStr=fixdt(1,32,16)
  IQN x IQN : tiiqmathlib/IQN x IQN  multiplyOption=Multiply
  Kx : Outport
  wires:
  Constant2/1 -> IQN x IQN/2
  x/1 -> IQN x IQN/1
  IQN x IQN/1 -> Kx/1

== system Final_V620140905h5b_fuben1/Subsystem1/ION multiply7 ==
  x : Inport
  Constant2 : Constant  Value=x  OutDataTypeStr=fixdt(1,32,16)
  IQN x IQN : tiiqmathlib/IQN x IQN  multiplyOption=Multiply
  Kx : Outport
  wires:
  IQN x IQN/1 -> Kx/1
  x/1 -> IQN x IQN/1
  Constant2/1 -> IQN x IQN/2

== system Final_V620140905h5b_fuben1/Subsystem2/ION multiply1 ==
  x : Inport
  Constant2 : Constant  Value=x  OutDataTypeStr=fixdt(1,32,16)
  IQN x IQN : tiiqmathlib/IQN x IQN  multiplyOption=Multiply
  Kx : Outport
  wires:
  Constant2/1 -> IQN x IQN/2
  x/1 -> IQN x IQN/1
  IQN x IQN/1 -> Kx/1

== system Final_V620140905h5b_fuben1/Subsystem2/ION multiply2 ==
  x : Inport
  Constant2 : Constant  Value=x  OutDataTypeStr=fixdt(1,32,16)
  IQN x IQN : tiiqmathlib/IQN x IQN  multiplyOption=Multiply
  Kx : Outport
  wires:
  Constant2/1 -> IQN x IQN/2
  x/1 -> IQN x IQN/1
  IQN x IQN/1 -> Kx/1

== system Final_V620140905h5b_fuben1/Subsystem2/ION multiply3 ==
  x : Inport
  Constant2 : Constant  Value=x  OutDataTypeStr=fixdt(1,32,16)
  IQN x IQN : tiiqmathlib/IQN x IQN  multiplyOption=Multiply
  Kx : Outport
  wires:
  IQN x IQN/1 -> Kx/1
  x/1 -> IQN x IQN/1
  Constant2/1 -> IQN x IQN/2

== system Final_V620140905h5b_fuben1/Subsystem2/ION multiply4 ==
  x : Inport
  Constant2 : Constant  Value=x  OutDataTypeStr=fixdt(1,32,16)
  IQN x IQN : tiiqmathlib/IQN x IQN  multiplyOption=Multiply
  Kx : Outport
  wires:
  Constant2/1 -> IQN x IQN/2
  x/1 -> IQN x IQN/1
  IQN x IQN/1 -> Kx/1

== system Final_V620140905h5b_fuben1/Subsystem2/ION multiply42 ==
  x : Inport
  Constant2 : Constant  Value=x  OutDataTypeStr=fixdt(1,32,16)
  IQN x IQN : tiiqmathlib/IQN x IQN  multiplyOption=Multiply
  Kx : Outport
  wires:
  IQN x IQN/1 -> Kx/1
  x/1 -> IQN x IQN/1
  Constant2/1 -> IQN x IQN/2

== system Final_V620140905h5b_fuben1/Subsystem2/ION multiply5 ==
  x : Inport
  Constant2 : Constant  Value=x  OutDataTypeStr=fixdt(1,32,16)
  IQN x IQN : tiiqmathlib/IQN x IQN  multiplyOption=Multiply
  Kx : Outport
  wires:
  IQN x IQN/1 -> Kx/1
  x/1 -> IQN x IQN/1
  Constant2/1 -> IQN x IQN/2

== system Final_V620140905h5b_fuben1/Subsystem3/ION multiply1 ==
  x : Inport
  Constant2 : Constant  Value=x  OutDataTypeStr=fixdt(1,32,16)
  IQN x IQN : tiiqmathlib/IQN x IQN  multiplyOption=Multiply
  Kx : Outport
  wires:
  IQN x IQN/1 -> Kx/1
  x/1 -> IQN x IQN/1
  Constant2/1 -> IQN x IQN/2

== system Final_V620140905h5b_fuben1/Subsystem3/ION multiply2 ==
  x : Inport
  Constant2 : Constant  Value=x  OutDataTypeStr=fixdt(1,32,16)
  IQN x IQN : tiiqmathlib/IQN x IQN  multiplyOption=Multiply
  Kx : Outport
  wires:
  Constant2/1 -> IQN x IQN/2
  x/1 -> IQN x IQN/1
  IQN x IQN/1 -> Kx/1

== system Final_V620140905h5b_fuben1/Subsystem3/ION multiply3 ==
  x : Inport
  Constant2 : Constant  Value=x  OutDataTypeStr=fixdt(1,32,16)
  IQN x IQN : tiiqmathlib/IQN x IQN  multiplyOption=Multiply
  Kx : Outport
  wires:
  IQN x IQN/1 -> Kx/1
  x/1 -> IQN x IQN/1
  Constant2/1 -> IQN x IQN/2

== system Final_V620140905h5b_fuben1/Subsystem3/ION multiply4 ==
  x : Inport
  Constant2 : Constant  Value=x  OutDataTypeStr=fixdt(1,32,16)
  IQN x IQN : tiiqmathlib/IQN x IQN  multiplyOption=Multiply
  Kx : Outport
  wires:
  Constant2/1 -> IQN x IQN/2
  x/1 -> IQN x IQN/1
  IQN x IQN/1 -> Kx/1

== system Final_V620140905h5b_fuben1/Subsystem3/ION multiply5 ==
  x : Inport
  Constant2 : Constant  Value=x  OutDataTypeStr=fixdt(1,32,16)
  IQN x IQN : tiiqmathlib/IQN x IQN  multiplyOption=Multiply
  Kx : Outport
  wires:
  IQN x IQN/1 -> Kx/1
  x/1 -> IQN x IQN/1
  Constant2/1 -> IQN x IQN/2

== system Final_V620140905h5b_fuben1/Subsystem4/If Action Subsystem ==
  Action Port : ActionPort  ActionType=then
  Constant4 : Constant  Value=0  OutDataTypeStr=int16
  Out1 : Outport
  wires:
  Constant4/1 -> Out1/1

== system Final_V620140905h5b_fuben1/Subsystem4/If Action Subsystem1 ==
  Action Port : ActionPort  ActionType=elseif
  Constant4 : Constant  OutDataTypeStr=int16
  Out1 : Outport
  wires:
  Constant4/1 -> Out1/1

== system Final_V620140905h5b_fuben1/Subsystem4/If Action Subsystem10 ==
  Action Port : ActionPort  ActionType=elseif
  Constant4 : Constant  Value=6  OutDataTypeStr=int16
  Out1 : Outport
  wires:
  Constant4/1 -> Out1/1

== system Final_V620140905h5b_fuben1/Subsystem4/If Action Subsystem11 ==
  Action Port : ActionPort  ActionType=elseif
  Constant4 : Constant  Value=7  OutDataTypeStr=int16
  Out1 : Outport
  wires:
  Constant4/1 -> Out1/1

== system Final_V620140905h5b_fuben1/Subsystem4/If Action Subsystem12 ==
  Action Port : ActionPort  ActionType=elseif
  Constant4 : Constant  OutDataTypeStr=int16
  Out1 : Outport
  wires:
  Constant4/1 -> Out1/1

== system Final_V620140905h5b_fuben1/Subsystem4/If Action Subsystem13 ==
  Action Port : ActionPort  ActionType=elseif
  Constant4 : Constant  Value=10  OutDataTypeStr=int16
  Out1 : Outport
  wires:
  Constant4/1 -> Out1/1

== system Final_V620140905h5b_fuben1/Subsystem4/If Action Subsystem14 ==
  Action Port : ActionPort  ActionType=elseif
  Constant4 : Constant  Value=11  OutDataTypeStr=int16
  Out1 : Outport
  wires:
  Constant4/1 -> Out1/1

== system Final_V620140905h5b_fuben1/Subsystem4/If Action Subsystem15 ==
  Action Port : ActionPort  ActionType=elseif
  Constant4 : Constant  Value=5  OutDataTypeStr=int16
  Out1 : Outport
  wires:
  Constant4/1 -> Out1/1

== system Final_V620140905h5b_fuben1/Subsystem4/If Action Subsystem2 ==
  Action Port : ActionPort  ActionType=elseif
  Constant4 : Constant  Value=10  OutDataTypeStr=int16
  Out1 : Outport
  wires:
  Constant4/1 -> Out1/1

== system Final_V620140905h5b_fuben1/Subsystem4/If Action Subsystem3 ==
  Action Port : ActionPort  ActionType=elseif
  Constant4 : Constant  Value=11  OutDataTypeStr=int16
  Out1 : Outport
  wires:
  Constant4/1 -> Out1/1

== system Final_V620140905h5b_fuben1/Subsystem4/If Action Subsystem4 ==
  Action Port : ActionPort  ActionType=elseif
  Constant4 : Constant  Value=6  OutDataTypeStr=int16
  Out1 : Outport
  wires:
  Constant4/1 -> Out1/1

== system Final_V620140905h5b_fuben1/Subsystem4/If Action Subsystem5 ==
  Action Port : ActionPort  ActionType=elseif
  Constant4 : Constant  Value=7  OutDataTypeStr=int16
  Out1 : Outport
  wires:
  Constant4/1 -> Out1/1

== system Final_V620140905h5b_fuben1/Subsystem4/If Action Subsystem6 ==
  Action Port : ActionPort  ActionType=elseif
  Constant4 : Constant  Value=4  OutDataTypeStr=int16
  Out1 : Outport
  wires:
  Constant4/1 -> Out1/1

== system Final_V620140905h5b_fuben1/Subsystem4/If Action Subsystem7 ==
  Action Port : ActionPort  ActionType=elseif
  Constant4 : Constant  Value=4  OutDataTypeStr=int16
  Out1 : Outport
  wires:
  Constant4/1 -> Out1/1

== system Final_V620140905h5b_fuben1/Subsystem4/If Action Subsystem8 ==
  Action Port : ActionPort  ActionType=elseif
  Constant4 : Constant  Value=2  OutDataTypeStr=int16
  Out1 : Outport
  wires:
  Constant4/1 -> Out1/1

== system Final_V620140905h5b_fuben1/Subsystem4/If Action Subsystem9 ==
  Action Port : ActionPort  ActionType=elseif
  Constant4 : Constant  Value=3  OutDataTypeStr=int16
  Out1 : Outport
  wires:
  Constant4/1 -> Out1/1
